simulink model "Quaternions_Method_merge_gio"  (R2021b)
settings: Solver=FixedStepAuto  StartTime=0.0  StopTime=Time  FixedStep=1e-3  RelTol=1e-13  AbsTol=1e-8
values from neighbouring files (symbols this model uses):
  a = 8.6251e+06    (= 8625100)    [Main.m]
  A_BN_0 = [1/3, 2/3, 2/3;             2/3, 1/3, -2/3;            -2/3, 2/3,-1/3]    [Main.m]
  A_rw = [1 0 0 1/sqrt(3);         0 1 0 1/sqrt(3) ... (first row only)    [Main.m]
  A_rw_star = [5/6 -1/6 -1/6;              -1/6  5/6 -1/6 ... (first row only)    [Main.m]
  c = 299792*10^3    (= 299792000)    [Main.m]
  e = 0.1195    [Main.m]
  f_mag = 5    [Main.m]
  G = [gn, gm, gvali, gsvi]    [Main.m]
  H = [hn, hm, hvali, hsvi]    [Main.m]
  H_0 = sqrt((g_1_0)^2 + (g_1_1)^2 + (h_1_1)^2)    [Main.m]
  i = 0.3815    [Main.m]
  MB = [2000; 0.3; 1; 0.12].*1e-2    [Main.m]
  mr = 1.2*1e-4    (= 0.00012)    [Main.m]
  muP = G*Mt    (= 398527110340000)    [Main.m]
  omega_0 = [om_x, om_y, om_z]    [Main.m]
  p_acc = deg2rad(5)    [Main.m]
  RD = 0.1*ones(1,10)    [Main.m]
  rho_d_MB = 0.1    [Main.m]
  rho_s_MB = 0.5    [Main.m]
  RS_MB = 0.5    [Main.m]
  RS_SP = 0.1    [Main.m]
  sig_b = sig_b^2    [Main.m]
  sig_n = 0.15*pi/180/3600/sqrt(t_sample)    [Main.m]
  SP = [2000; 0.3; 1; 0.12].*1e-2    [Main.m]
  T = 2*pi/n    [Main.m]
  t_sample = 1/5    (= 0.2)    [Main.m]
  theta0 = 0    [Main.m]
  w_E = (2*pi)/(24*3600)    (= 7.27220521664e-05)    [Main.m]
undefined symbols (not defined in the file or in its folder): magnitude
libraries: matrix_library x18, vrlib x8, simulink x2, simulink_extras x1
(part 5 of 6)

== system Quaternions_Method_merge_gio/Enviroment/Solar Radiation Perturbation/Torque_arm/creazione raggi vettore tra CM MB e centro facce illuminate della faccia che ha come normale l'asse j/If Action Subsystem1 ==
  Areas_vect : Inport
  MB : Inport  Port=2
  Action Port : ActionPort  ActionPortLabel=if(u1<0 & u2>0)
  Add : Sum  Inputs=+|-
  Add1 : Sum  Inputs=+|-
  Add2 : Sum
  Demux : Demux  Outputs=3
  Demux2 : Demux
  Divide : Product  Inputs=*/
  Divide1 : Product  Inputs=*/
  Gain{,1..3} (4 alike) : Gain  Gain=1/2
  Gain4 : Gain  Gain=-1
  Ground : Ground
  Ground1 : Ground
  Mux : Mux  Inputs=3
  Mux1 : Mux  Inputs=3
  Reshape : Reshape  OutputDimensionality=Column vector (2-D)
  Reshape2 : Reshape  OutputDimensionality=Column vector (2-D)
  Reshape3 : Reshape  OutputDimensionality=Column vector (2-D)
  Terminator{1..2,8..9} (4 alike) : Terminator
  r_cface_cluce_x_pos_z_neg : Outport
  wires:
  Demux/3 -> Terminator8/1
  Demux/1 -> Terminator9/1
  Add2/1 -> r_cface_cluce_x_pos_z_neg/1
  Reshape3/1 -> Add2/2
  Reshape2/1 -> Add2/1
  [a_MB] -> Gain2/1
  Divide1/1 -> Gain3/1
  Gain2/1 -> Add1/1
  Gain3/1 -> Add1/2
  Ground/1 -> Mux1/3, Mux1/2
  Mux1/1 -> Reshape3/1  "raggio vettore che collega il centro geom della faccia con il centro geom della faccia illuminata dal sole lungo i"
  [h_MB] -> Divide1/2
  Add1/1 -> Mux1/1
  Reshape/1 -> Demux/1
  Ground1/1 -> Mux/1, Mux/2
  Areas_vect/1 -> Reshape/1
  [a_MB] -> Divide/2
  Gain/1 -> Add/1
  [h_MB] -> Gain/1
  Demux/2 -> Divide/1, Divide1/1
  Gain1/1 -> Add/2
  Mux/1 -> Reshape2/1  "raggio vettore che collega il centro geom della faccia con il centro geom della faccia illuminata dal sole lungo -k"
  Divide/1 -> Gain1/1
  Add/1 -> Gain4/1
  Gain4/1 -> Mux/3
  Demux2/1 -> Terminator2/1
  Demux2/2 -> [a_MB]
  MB/1 -> Demux2/1
  Demux2/3 -> Terminator1/1
  Demux2/4 -> [h_MB]

== system Quaternions_Method_merge_gio/Enviroment/Solar Radiation Perturbation/Torque_arm/creazione raggi vettore tra CM MB e centro facce illuminate della faccia che ha come normale l'asse j/If Action Subsystem2 ==
  Areas_vect : Inport
  MB : Inport  Port=2
  Action Port : ActionPort  ActionPortLabel=if(u1>0 & u2<0)
  Add : Sum  Inputs=+|-
  Add1 : Sum  Inputs=+|-
  Add2 : Sum
  Demux : Demux  Outputs=3
  Demux2 : Demux
  Divide : Product  Inputs=*/
  Divide1 : Product  Inputs=*/
  Gain{,1..3} (4 alike) : Gain  Gain=1/2
  Gain4 : Gain  Gain=-1
  Ground : Ground
  Ground1 : Ground
  Mux : Mux  Inputs=3
  Mux1 : Mux  Inputs=3
  Reshape : Reshape  OutputDimensionality=Column vector (2-D)
  Reshape2 : Reshape  OutputDimensionality=Column vector (2-D)
  Reshape3 : Reshape  OutputDimensionality=Column vector (2-D)
  Terminator{1..2,8..9} (4 alike) : Terminator
  r_cface_cluce_x_neg_z_pos : Outport
  wires:
  Add/1 -> Mux/3
  Divide/1 -> Gain1/1
  Mux/1 -> Reshape2/1  "raggio vettore che collega il centro geom della faccia con il centro geom della faccia illuminata dal sole lungo k"
  Gain1/1 -> Add/2
  Demux/2 -> Divide1/1, Divide/1
  [h_MB] -> Gain/1
  Gain/1 -> Add/1
  [a_MB] -> Divide/2
  Areas_vect/1 -> Reshape/1
  Ground1/1 -> Mux/2, Mux/1
  Reshape/1 -> Demux/1
  [h_MB] -> Divide1/2
  Mux1/1 -> Reshape3/1  "raggio vettore che collega il centro geom della faccia con il centro geom della faccia illuminata dal sole lungo -i"
  Ground/1 -> Mux1/2, Mux1/3
  Gain3/1 -> Add1/2
  Gain2/1 -> Add1/1
  Divide1/1 -> Gain3/1
  [a_MB] -> Gain2/1
  Reshape2/1 -> Add2/1
  Reshape3/1 -> Add2/2
  Add2/1 -> r_cface_cluce_x_neg_z_pos/1
  Demux/1 -> Terminator9/1
  Demux/3 -> Terminator8/1
  Gain4/1 -> Mux1/1
  Add1/1 -> Gain4/1
  Demux2/1 -> Terminator2/1
  Demux2/2 -> [a_MB]
  MB/1 -> Demux2/1
  Demux2/3 -> Terminator1/1
  Demux2/4 -> [h_MB]

== system Quaternions_Method_merge_gio/Enviroment/Solar Radiation Perturbation/Torque_arm/creazione raggi vettore tra CM MB e centro facce illuminate della faccia che ha come normale l'asse j/If Action Subsystem3 ==
  Areas_vect : Inport
  MB : Inport  Port=2
  Action Port : ActionPort  ActionPortLabel=if(u1<0 & u2<0)
  Add : Sum  Inputs=+|-
  Add1 : Sum  Inputs=+|-
  Add2 : Sum
  Demux : Demux  Outputs=3
  Demux2 : Demux
  Divide : Product  Inputs=*/
  Divide1 : Product  Inputs=*/
  Gain{,1..3} (4 alike) : Gain  Gain=1/2
  Gain4 : Gain  Gain=-1
  Gain5 : Gain  Gain=-1
  Ground : Ground
  Ground1 : Ground
  Mux : Mux  Inputs=3
  Mux1 : Mux  Inputs=3
  Reshape : Reshape  OutputDimensionality=Column vector (2-D)
  Reshape2 : Reshape  OutputDimensionality=Column vector (2-D)
  Reshape3 : Reshape  OutputDimensionality=Column vector (2-D)
  Terminator{1..2,8..9} (4 alike) : Terminator
  r_cface_cluce_x_neg_z_neg : Outport
  wires:
  Add1/1 -> Gain4/1
  Gain4/1 -> Mux1/1
  Demux/3 -> Terminator8/1
  Demux/1 -> Terminator9/1
  Add2/1 -> r_cface_cluce_x_neg_z_neg/1
  Reshape3/1 -> Add2/2
  Reshape2/1 -> Add2/1
  [a_MB] -> Gain2/1
  Divide1/1 -> Gain3/1
  Gain2/1 -> Add1/1
  Gain3/1 -> Add1/2
  Ground/1 -> Mux1/3, Mux1/2
  Mux1/1 -> Reshape3/1  "raggio vettore che collega il centro geom della faccia con il centro geom della faccia illuminata dal sole lungo -i"
  [h_MB] -> Divide1/2
  Reshape/1 -> Demux/1
  Ground1/1 -> Mux/1, Mux/2
  Areas_vect/1 -> Reshape/1
  [a_MB] -> Divide/2
  Gain/1 -> Add/1
  [h_MB] -> Gain/1
  Demux/2 -> Divide/1, Divide1/1
  Gain1/1 -> Add/2
  Mux/1 -> Reshape2/1  "raggio vettore che collega il centro geom della faccia con il centro geom della faccia illuminata dal sole lungo -k"
  Divide/1 -> Gain1/1
  Add/1 -> Gain5/1
  Gain5/1 -> Mux/3
  Demux2/1 -> Terminator2/1
  Demux2/2 -> [a_MB]
  MB/1 -> Demux2/1
  Demux2/3 -> Terminator1/1
  Demux2/4 -> [h_MB]

== system Quaternions_Method_merge_gio/Enviroment/Solar Radiation Perturbation/Torque_arm/creazione raggi vettore tra CM MB e centro facce illuminate della faccia che ha come normale l'asse j/If Action Subsystem4 ==
  Action Port : ActionPort  ActionPortLabel=else
  Constant : Constant  Value=[0;0;0]
  Out1 : Outport
  wires:
  Constant/1 -> Out1/1

== system Quaternions_Method_merge_gio/Enviroment/Solar Radiation Perturbation/Torque_arm/creazione raggi vettore tra CM MB e centro facce illuminate della faccia che ha come normale l'asse j/If Action Subsystem5 ==
  Action Port : ActionPort  ActionPortLabel=else
  Constant : Constant  Value=[0;0;0]
  Out1 : Outport
  wires:
  Constant/1 -> Out1/1

== system Quaternions_Method_merge_gio/Enviroment/Solar Radiation Perturbation/Torque_arm/creazione raggi vettore tra CM MB e centro facce illuminate della faccia che ha come normale l'asse j/If Action Subsystem6 ==
  Action Port : ActionPort  ActionPortLabel=else
  Constant : Constant  Value=[0;0;0]
  Out1 : Outport
  wires:
  Constant/1 -> Out1/1

== system Quaternions_Method_merge_gio/Enviroment/Solar Radiation Perturbation/Torque_arm/creazione raggi vettore tra CM MB e centro facce illuminate della faccia che ha come normale l'asse j/If Action Subsystem7 ==
  Action Port : ActionPort  ActionPortLabel=else
  Constant : Constant  Value=[0;0;0]
  Out1 : Outport
  wires:
  Constant/1 -> Out1/1

== system Quaternions_Method_merge_gio/Enviroment/Solar Radiation Perturbation/Torque_arm/creazione raggi vettore tra CM MB e centro facce illuminate della faccia che ha come normale l'asse j/creating distance between cm MB and centro geom lato1 ==
  MB : Inport
  pointer : Inport  Port=2
  Demux : Demux
  Ground : Ground
  Mux : Mux  Inputs=3
  Product : Product
  Reshape : Reshape  OutputDimensionality=Column vector (2-D)
  Terminator : Terminator
  Terminator1 : Terminator
  Terminator2 : Terminator
  Out1 : Outport
  wires:
  Reshape/1 -> Out1/1
  Mux/1 -> Reshape/1
  MB/1 -> Demux/1
  Demux/1 -> Terminator/1
  Demux/2 -> Terminator1/1
  Demux/3 -> Terminator2/1
  Ground/1 -> Mux/2, Mux/1
  Demux/4 -> Product/1
  pointer/1 -> Product/2
  Product/1 -> Mux/3

== system Quaternions_Method_merge_gio/Enviroment/Solar Radiation Perturbation/Torque_arm/creazione raggi vettore tra CM MB e centro facce illuminate della faccia che ha come normale l'asse k/If Action Subsystem ==
  Areas_vect : Inport
  MB : Inport  Port=2
  Action Port : ActionPort  ActionPortLabel=if(u1>0 & u2>0)
  Add : Sum  Inputs=+|-
  Add1 : Sum  Inputs=+|-
  Add2 : Sum
  Demux : Demux  Outputs=3
  Demux1 : Demux  Outputs=3
  Demux2 : Demux
  Divide : Product  Inputs=*/
  Divide1 : Product  Inputs=*/
  Gain{,1..3} (4 alike) : Gain  Gain=1/2
  Ground : Ground
  Ground1 : Ground
  Mux : Mux  Inputs=3
  Mux1 : Mux  Inputs=3
  Reshape{,1..3} (4 alike) : Reshape  OutputDimensionality=Column vector (2-D)
  Terminator{,1..3,8..9} (6 alike) : Terminator
  r_cface_cluce_xy_pos : Outport
  wires:
  Add/1 -> Mux/2
  Divide/1 -> Gain1/1
  Mux/1 -> Reshape2/1  "raggio vettore che collega il centro geom della faccia con il centro geom della faccia illuminata dal sole lungo j"
  Gain1/1 -> Add/2
  Demux/3 -> Divide/1
  [b_MB] -> Gain/1
  Gain/1 -> Add/1
  [a_MB] -> Divide/2
  Areas_vect/1 -> Reshape/1, Reshape1/1
  Ground1/1 -> Mux/1, Mux/3
  Reshape/1 -> Demux/1
  Add1/1 -> Mux1/1
  [b_MB] -> Divide1/2
  Mux1/1 -> Reshape3/1  "raggio vettore che collega il centro geom della faccia con il centro geom della faccia illuminata dal sole lungo x"
  Ground/1 -> Mux1/2, Mux1/3
  Demux1/3 -> Divide1/1
  Gain3/1 -> Add1/2
  Gain2/1 -> Add1/1
  Reshape1/1 -> Demux1/1
  Divide1/1 -> Gain3/1
  [a_MB] -> Gain2/1
  Reshape2/1 -> Add2/1
  Reshape3/1 -> Add2/2
  Add2/1 -> r_cface_cluce_xy_pos/1
  Demux1/1 -> Terminator/1
  Demux1/2 -> Terminator1/1
  Demux/1 -> Terminator9/1
  Demux/2 -> Terminator8/1
  MB/1 -> Demux2/1
  Demux2/1 -> Terminator2/1
  Demux2/2 -> [a_MB]
  Demux2/3 -> [b_MB]
  Demux2/4 -> Terminator3/1

== system Quaternions_Method_merge_gio/Enviroment/Solar Radiation Perturbation/Torque_arm/creazione raggi vettore tra CM MB e centro facce illuminate della faccia che ha come normale l'asse k/If Action Subsystem1 ==
  Areas_vect : Inport
  MB : Inport  Port=2
  Action Port : ActionPort  ActionPortLabel=if(u1>0 & u2<0)
  Add : Sum  Inputs=+|-
  Add1 : Sum  Inputs=+|-
  Add2 : Sum
  Demux : Demux  Outputs=3
  Demux1 : Demux  Outputs=3
  Demux2 : Demux
  Divide : Product  Inputs=*/
  Divide1 : Product  Inputs=*/
  Gain{,1..3} (4 alike) : Gain  Gain=1/2
  Gain4 : Gain  Gain=-1
  Ground : Ground
  Ground1 : Ground
  Mux : Mux  Inputs=3
  Mux1 : Mux  Inputs=3
  Reshape{,1..3} (4 alike) : Reshape  OutputDimensionality=Column vector (2-D)
  Terminator{,1..3,8..9} (6 alike) : Terminator
  r_cface_cluce_xpos_y_neg : Outport
  wires:
  Add/1 -> Gain4/1
  Divide/1 -> Gain1/1
  Mux/1 -> Reshape2/1  "raggio vettore che collega il centro geom della faccia con il centro geom della faccia illuminata dal sole lungo -j"
  Gain1/1 -> Add/2
  Demux/3 -> Divide/1
  Gain/1 -> Add/1
  Areas_vect/1 -> Reshape/1, Reshape1/1
  Ground1/1 -> Mux/1, Mux/3
  Reshape/1 -> Demux/1
  Mux1/1 -> Reshape3/1  "raggio vettore che collega il centro geom della faccia con il centro geom della faccia illuminata dal sole lungo i"
  Ground/1 -> Mux1/2, Mux1/3
  Demux1/3 -> Divide1/1
  Gain3/1 -> Add1/2
  Gain2/1 -> Add1/1
  Reshape1/1 -> Demux1/1
  Divide1/1 -> Gain3/1
  Reshape2/1 -> Add2/1
  Reshape3/1 -> Add2/2
  Add2/1 -> r_cface_cluce_xpos_y_neg/1
  Demux1/1 -> Terminator/1
  Demux1/2 -> Terminator1/1
  Demux/1 -> Terminator9/1
  Demux/2 -> Terminator8/1
  Gain4/1 -> Mux/2
  [a_MB] -> Divide/2
  [b_MB] -> Gain/1
  Add1/1 -> Mux1/1
  [b_MB] -> Divide1/2
  [a_MB] -> Gain2/1
  Demux2/1 -> Terminator2/1
  Demux2/2 -> [a_MB]
  MB/1 -> Demux2/1
  Demux2/3 -> [b_MB]
  Demux2/4 -> Terminator3/1

== system Quaternions_Method_merge_gio/Enviroment/Solar Radiation Perturbation/Torque_arm/creazione raggi vettore tra CM MB e centro facce illuminate della faccia che ha come normale l'asse k/If Action Subsystem2 ==
  Areas_vect : Inport
  MB1 : Inport  Port=2
  Action Port : ActionPort  ActionPortLabel=if(u1<0 & u2<0)
  Add : Sum  Inputs=+|-
  Add1 : Sum  Inputs=+|-
  Add2 : Sum
  Demux : Demux  Outputs=3
  Demux1 : Demux  Outputs=3
  Demux2 : Demux
  Divide : Product  Inputs=*/
  Divide1 : Product  Inputs=*/
  Gain{,1..3} (4 alike) : Gain  Gain=1/2
  Gain4 : Gain  Gain=-1
  Gain5 : Gain  Gain=-1
  Ground : Ground
  Ground1 : Ground
  Mux : Mux  Inputs=3
  Mux1 : Mux  Inputs=3
  Reshape{,1..3} (4 alike) : Reshape  OutputDimensionality=Column vector (2-D)
  Terminator{,1..3,8..9} (6 alike) : Terminator
  r_cface_cluce_xneg_y_neg : Outport
  wires:
  [a_MB] -> Divide1/2
  [b_MB] -> Gain2/1
  Add1/1 -> Gain5/1
  Gain4/1 -> Mux/1
  Add/1 -> Gain4/1
  [a_MB] -> Gain/1
  [b_MB] -> Divide/2
  Divide/1 -> Gain1/1
  Mux/1 -> Reshape2/1  "raggio vettore che collega il centro geom della faccia con il centro geom della faccia illuminata dal sole lungo -i"
  Gain1/1 -> Add/2
  Demux/3 -> Divide/1
  Gain/1 -> Add/1
  Areas_vect/1 -> Reshape/1, Reshape1/1
  Ground1/1 -> Mux/3, Mux/2
  Reshape/1 -> Demux/1
  Mux1/1 -> Reshape3/1  "raggio vettore che collega il centro geom della faccia con il centro geom della faccia illuminata dal sole lungo -j"
  Ground/1 -> Mux1/3, Mux1/1
  Demux1/3 -> Divide1/1
  Gain3/1 -> Add1/2
  Gain2/1 -> Add1/1
  Reshape1/1 -> Demux1/1
  Divide1/1 -> Gain3/1
  Reshape2/1 -> Add2/1
  Reshape3/1 -> Add2/2
  Add2/1 -> r_cface_cluce_xneg_y_neg/1
  Demux1/1 -> Terminator/1
  Demux1/2 -> Terminator1/1
  Demux/1 -> Terminator9/1
  Demux/2 -> Terminator8/1
  Gain5/1 -> Mux1/2
  Demux2/1 -> Terminator2/1
  Demux2/2 -> [a_MB]
  MB1/1 -> Demux2/1
  Demux2/3 -> [b_MB]
  Demux2/4 -> Terminator3/1

== system Quaternions_Method_merge_gio/Enviroment/Solar Radiation Perturbation/Torque_arm/creazione raggi vettore tra CM MB e centro facce illuminate della faccia che ha come normale l'asse k/If Action Subsystem3 ==
  Action Port : ActionPort  ActionPortLabel=else
  Constant : Constant  Value=[0;0;0]
  Out1 : Outport
  wires:
  Constant/1 -> Out1/1

== system Quaternions_Method_merge_gio/Enviroment/Solar Radiation Perturbation/Torque_arm/creazione raggi vettore tra CM MB e centro facce illuminate della faccia che ha come normale l'asse k/If Action Subsystem4 ==
  Areas_vect : Inport
  MB1 : Inport  Port=2
  Action Port : ActionPort  ActionPortLabel=if(u1<0 & u2>0)
  Add : Sum  Inputs=+|-
  Add1 : Sum  Inputs=+|-
  Add2 : Sum
  Demux : Demux  Outputs=3
  Demux1 : Demux  Outputs=3
  Demux2 : Demux
  Divide : Product  Inputs=*/
  Divide1 : Product  Inputs=*/
  Gain{,1..3} (4 alike) : Gain  Gain=1/2
  Gain4 : Gain  Gain=-1
  Ground : Ground
  Ground1 : Ground
  Mux : Mux  Inputs=3
  Mux1 : Mux  Inputs=3
  Reshape{,1..3} (4 alike) : Reshape  OutputDimensionality=Column vector (2-D)
  Terminator{,1..3,8..9} (6 alike) : Terminator
  r_cface_cluce_xneg_y_pos : Outport
  wires:
  Demux/2 -> Terminator8/1
  Demux/1 -> Terminator9/1
  Demux1/2 -> Terminator1/1
  Demux1/1 -> Terminator/1
  Add2/1 -> r_cface_cluce_xneg_y_pos/1
  Reshape3/1 -> Add2/2
  Reshape2/1 -> Add2/1
  Divide1/1 -> Gain3/1
  Reshape1/1 -> Demux1/1
  Gain2/1 -> Add1/1
  Gain3/1 -> Add1/2
  Demux1/3 -> Divide1/1
  Ground/1 -> Mux1/1, Mux1/3
  Mux1/1 -> Reshape3/1  "raggio vettore che collega il centro geom della faccia con il centro geom della faccia illuminata dal sole lungo j"
  Reshape/1 -> Demux/1
  Ground1/1 -> Mux/2, Mux/3
  Areas_vect/1 -> Reshape1/1, Reshape/1
  Gain/1 -> Add/1
  Demux/3 -> Divide/1
  Gain1/1 -> Add/2
  Mux/1 -> Reshape2/1  "raggio vettore che collega il centro geom della faccia con il centro geom della faccia illuminata dal sole lungo -i"
  Divide/1 -> Gain1/1
  [b_MB] -> Divide/2
  [a_MB] -> Gain/1
  Add/1 -> Gain4/1
  Gain4/1 -> Mux/1
  Add1/1 -> Mux1/2
  [b_MB] -> Gain2/1
  [a_MB] -> Divide1/2
  Demux2/1 -> Terminator2/1
  Demux2/2 -> [a_MB]
  MB1/1 -> Demux2/1
  Demux2/3 -> [b_MB]
  Demux2/4 -> Terminator3/1

== system Quaternions_Method_merge_gio/Enviroment/Solar Radiation Perturbation/Torque_arm/creazione raggi vettore tra CM MB e centro facce illuminate della faccia che ha come normale l'asse k/If Action Subsystem5 ==
  Action Port : ActionPort  ActionPortLabel=else
  Constant : Constant  Value=[0;0;0]
  Out1 : Outport
  wires:
  Constant/1 -> Out1/1

== system Quaternions_Method_merge_gio/Enviroment/Solar Radiation Perturbation/Torque_arm/creazione raggi vettore tra CM MB e centro facce illuminate della faccia che ha come normale l'asse k/If Action Subsystem6 ==
  Action Port : ActionPort  ActionPortLabel=else
  Constant : Constant  Value=[0;0;0]
  Out1 : Outport
  wires:
  Constant/1 -> Out1/1

== system Quaternions_Method_merge_gio/Enviroment/Solar Radiation Perturbation/Torque_arm/creazione raggi vettore tra CM MB e centro facce illuminate della faccia che ha come normale l'asse k/If Action Subsystem7 ==
  Action Port : ActionPort  ActionPortLabel=else
  Constant : Constant  Value=[0;0;0]
  Out1 : Outport
  wires:
  Constant/1 -> Out1/1

== system Quaternions_Method_merge_gio/Enviroment/Solar Radiation Perturbation/Torque_arm/creazione raggi vettore tra CM MB e centro facce illuminate della faccia che ha come normale l'asse k/creating distance between cm MB and centro geom lato1 ==
  MB : Inport
  pointer : Inport  Port=2
  Demux : Demux
  Ground : Ground
  Mux : Mux  Inputs=3
  Product : Product
  Reshape : Reshape  OutputDimensionality=Column vector (2-D)
  Terminator : Terminator
  Terminator2 : Terminator
  Terminator3 : Terminator
  Out1 : Outport
  wires:
  Reshape/1 -> Out1/1
  Mux/1 -> Reshape/1
  MB/1 -> Demux/1
  Demux/1 -> Terminator/1
  Demux/3 -> Terminator2/1
  Ground/1 -> Mux/3, Mux/2
  Demux/4 -> Terminator3/1
  Product/1 -> Mux/1
  pointer/1 -> Product/2
  Demux/2 -> Product/1

== system Quaternions_Method_merge_gio/Sensors/Magnetometer1/Magnetometer /Error Matrices/A_NonOrtho ==
  Constant : Constant
  Constant1 : Constant  Value=0
  Constant2 : Constant  Value=0
  Constant3 : Constant  Value=-0.04
  Constant4 : Constant
  Constant5 : Constant  Value=0
  Constant6 : Constant  Value=0.02
  Constant7 : Constant  Value=0.01
  Constant8 : Constant
  Reshape : Reshape  OutputDimensionality=Customize  OutputDimensions=[3,3]
  Vector Concatenate : Concatenate  NumInputs=9
  A_no : Outport
  wires:
  [A31] -> Vector Concatenate/3
  [A12] -> Vector Concatenate/4
  [A21] -> Vector Concatenate/2
  [A33] -> Vector Concatenate/9
  [A32] -> Vector Concatenate/6
  [A22] -> Vector Concatenate/5
  [A13] -> Vector Concatenate/7
  [A23] -> Vector Concatenate/8
  [A11] -> Vector Concatenate/1
  Vector Concatenate/1 -> Reshape/1
  Reshape/1 -> A_no/1
  Constant/1 -> [A11]
  Constant1/1 -> [A21]
  Constant2/1 -> [A31]
  Constant3/1 -> [A12]
  Constant4/1 -> [A22]
  Constant5/1 -> [A32]
  Constant6/1 -> [A13]
  Constant7/1 -> [A23]
  Constant8/1 -> [A33]

== system Quaternions_Method_merge_gio/Sensors/Magnetometer1/Magnetometer /Error Matrices/A_ScaleFactor ==
  Constant : Constant  Value=1.08
  Constant{1..2,4..7} (6 alike) : Constant  Value=0
  Constant3 : Constant  Value=0.95
  Constant8 : Constant  Value=1.10
  Reshape : Reshape  OutputDimensionality=Customize  OutputDimensions=[3,3]
  Vector Concatenate : Concatenate  NumInputs=9
  A_sf : Outport
  wires:
  [A31] -> Vector Concatenate/3
  [A12] -> Vector Concatenate/4
  [A21] -> Vector Concatenate/2
  [A33] -> Vector Concatenate/9
  [A32] -> Vector Concatenate/6
  [A22] -> Vector Concatenate/5
  [A13] -> Vector Concatenate/7
  [A23] -> Vector Concatenate/8
  [A11] -> Vector Concatenate/1
  Vector Concatenate/1 -> Reshape/1
  Reshape/1 -> A_sf/1
  Constant/1 -> [A11]
  Constant1/1 -> [A21]
  Constant2/1 -> [A31]
  Constant4/1 -> [A12]
  Constant3/1 -> [A22]
  Constant5/1 -> [A32]
  Constant6/1 -> [A13]
  Constant7/1 -> [A23]
  Constant8/1 -> [A33]

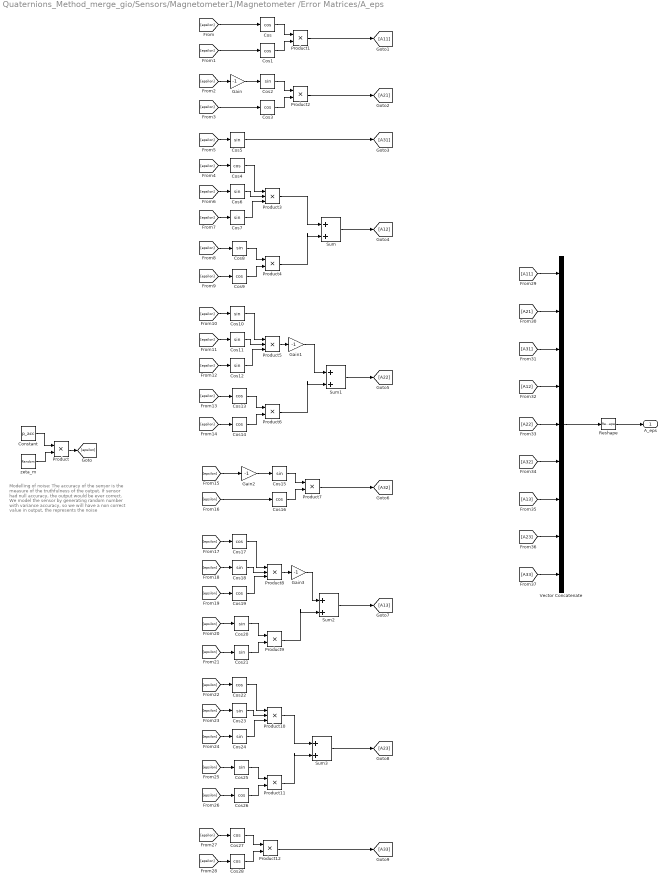
== system Quaternions_Method_merge_gio/Sensors/Magnetometer1/Magnetometer /Error Matrices/A_eps ==
  note: Modelling of noise: The accuracy of the sensor
      | is the measure of the truthfulness of the output.
      | If sensor had null accuracy, the output would be
      | ever correct. We model the  sensor by generating
      | random number with variance accuracy, so we
      | will have a non correct value in output, the
      | represents the noise
  Constant : Constant  Value=p_acc
  Cos{,1,3..4,9,13..14,16..17,19,22,26..28} (14 alike) : Trigonometry  Operator=cos
  Cos{2,5..8,10..12,15,18,20..21,23..25} (15 alike) : Trigonometry
  Gain{,1..3} (4 alike) : Gain  Gain=-1
  Product{,1..2,4,6..7,9,11..12} (9 alike) : Product
  Product{3,5,8,10} (4 alike) : Product  Inputs=3
  Reshape : Reshape  OutputDimensionality=Customize  OutputDimensions=[3,3]
  Sum{,1..3} (4 alike) : Sum  Inputs=|+|+|
  Vector Concatenate : Concatenate  NumInputs=9
  zeta_m : RandomNumber  Variance=p_acc  Seed=1  SampleTime=1/f_mag
  A_eps : Outport
  wires:
  Reshape/1 -> A_eps/1
  Vector Concatenate/1 -> Reshape/1
  Constant/1 -> Product/1
  zeta_m/1 -> Product/2
  Product/1 -> [epsilon]
  [epsilon] -> Cos/1
  [epsilon] -> Cos1/1
  Cos/1 -> Product1/1
  Cos1/1 -> Product1/2
  Product1/1 -> [A11]
  Cos2/1 -> Product2/1
  Cos3/1 -> Product2/2
  [epsilon] -> Cos3/1
  Product2/1 -> [A21]
  [epsilon] -> Gain/1
  Gain/1 -> Cos2/1
  [epsilon] -> Cos5/1
  Cos5/1 -> [A31]
  Cos4/1 -> Product3/1
  Cos6/1 -> Product3/2
  [epsilon] -> Cos4/1
  [epsilon] -> Cos6/1
  Product3/1 -> Sum/1
  [epsilon] -> Cos7/1
  Cos7/1 -> Product3/3
  [epsilon] -> Cos8/1
  Product4/1 -> Sum/2
  [epsilon] -> Cos9/1
  Cos9/1 -> Product4/2
  Cos8/1 -> Product4/1
  Sum/1 -> [A12]
  [epsilon] -> Cos11/1
  [epsilon] -> Cos10/1
  Cos11/1 -> Product5/2
  Cos10/1 -> Product5/1
  [epsilon] -> Cos13/1
  Sum1/1 -> [A22]
  Cos13/1 -> Product6/1
  [epsilon] -> Cos14/1
  Cos12/1 -> Product5/3
  Cos14/1 -> Product6/2
  Product6/1 -> Sum1/2
  [epsilon] -> Cos12/1
  Product5/1 -> Gain1/1
  Gain1/1 -> Sum1/1
  Gain2/1 -> Cos15/1
  [epsilon] -> Gain2/1
  Product7/1 -> [A32]
  Cos16/1 -> Product7/2
  Cos15/1 -> Product7/1
  [epsilon] -> Cos16/1
  Gain3/1 -> Sum2/1
  Product8/1 -> Gain3/1
  Cos18/1 -> Product8/2
  [epsilon] -> Cos18/1
  Sum2/1 -> [A13]
  Cos20/1 -> Product9/1
  Cos17/1 -> Product8/1
  [epsilon] -> Cos19/1
  Cos19/1 -> Product8/3
  Product9/1 -> Sum2/2
  [epsilon] -> Cos17/1
  Cos21/1 -> Product9/2
  [epsilon] -> Cos20/1
  [epsilon] -> Cos21/1
  [epsilon] -> Cos23/1
  [epsilon] -> Cos22/1
  Cos23/1 -> Product10/2
  Cos22/1 -> Product10/1
  [epsilon] -> Cos25/1
  Sum3/1 -> [A23]
  Cos25/1 -> Product11/1
  [epsilon] -> Cos26/1
  Product10/1 -> Sum3/1
  Cos24/1 -> Product10/3
  Cos26/1 -> Product11/2
  Product11/1 -> Sum3/2
  [epsilon] -> Cos24/1
  Cos27/1 -> Product12/1
  Cos28/1 -> Product12/2
  [epsilon] -> Cos27/1
  [epsilon] -> Cos28/1
  Product12/1 -> [A33]
  [A11] -> Vector Concatenate/1
  [A21] -> Vector Concatenate/2
  [A31] -> Vector Concatenate/3
  [A12] -> Vector Concatenate/4
  [A22] -> Vector Concatenate/5
  [A32] -> Vector Concatenate/6
  [A13] -> Vector Concatenate/7
  [A23] -> Vector Concatenate/8
  [A33] -> Vector Concatenate/9

== system Quaternions_Method_merge_gio/Sensors/Magnetometer1/b_B computation/Saturation/If Action Subsystem ==
  b_B : Inport
  Action Port : ActionPort  ActionPortLabel=if(u1 < mr)
  b_B* : Outport
  wires:
  b_B/1 -> b_B*/1

== system Quaternions_Method_merge_gio/Sensors/Magnetometer1/b_B computation/Saturation/If Action Subsystem1 ==
  mr : Inport
  b_B : Inport  Port=2
  Action Port : ActionPort  ActionPortLabel=else
  Normalize Vector : vrlib/Utilities/Normalize Vector  maxzero=0
  Product : Product
  b_B_sat : Outport
  wires:
  b_B/1 -> Normalize Vector/1
  Product/1 -> b_B_sat/1
  mr/1 -> Product/1
  Normalize Vector/1 -> Product/2

== system Quaternions_Method_merge_gio/Enviroment/Solar Radiation Perturbation/Sum forces/determine highlighted area/creazione della matrice che ha per colonne i vettori distanza tra il CM del MB e i centri geom delle aree illuminate dal sole /creazione raggi vettore tra CM MB e centro facce illuminate della faccia che ha come normale l'asse i ==
  S_B : Inport
  MB : Inport  Port=2
  A_vect : Inport  Port=3
  Add2 : Sum  Inputs=+|+|+|+|+
  Demux1 : Demux  Outputs=3
  If Action Subsystem : Subsystem  TreatAsAtomicUnit=on
  If Action Subsystem1 : Subsystem  TreatAsAtomicUnit=on
  If Action Subsystem2 : Subsystem  TreatAsAtomicUnit=on
  If Action Subsystem3 : Subsystem  TreatAsAtomicUnit=on
  If Action Subsystem4 : Subsystem  TreatAsAtomicUnit=on
  If Action Subsystem5 : Subsystem  TreatAsAtomicUnit=on
  If Action Subsystem6 : Subsystem  TreatAsAtomicUnit=on
  If Action Subsystem8 : Subsystem  TreatAsAtomicUnit=on
  If1 : If  NumInputs=2  IfExpression=u1>0 & u2>0
  If2 : If  NumInputs=2  IfExpression=u1<0 & u2>0
  If3 : If  NumInputs=2  IfExpression=u1>0 & u2<0
  If4 : If  NumInputs=2  IfExpression=u1<0 & u2<0
  Merge{,1..3} (4 alike) : Merge
  Reshape1 : Reshape  OutputDimensionality=Column vector (2-D)
  Terminator1 : Terminator
  creating distance between cm MB and centro geom lato : Subsystem
  Out1 : Outport
  wires:
  [A_vect] -> If Action Subsystem2/1(Areas_vect)
  [A_vect] -> If Action Subsystem1/1(Areas_vect)
  [A_vect] -> If Action Subsystem4/1(Areas_vect)
  Add2/1 -> Out1/1
  Merge3/1 -> Add2/5  "raggio vettore centro geom lato- centro geom lato illuminato"
  If4/1 -> If Action Subsystem2/Action
  If Action Subsystem2/1(r_cface_cluce_yneg_z_neg) -> Merge3/1
  If3/1 -> If Action Subsystem1/Action
  [A_vect] -> If Action Subsystem/1(Areas_vect)
  Merge1/1 -> Add2/3  "raggio vettore centro geom lato- centro geom lato illuminato"
  If Action Subsystem4/1(r_cface_cluce_zneg_y_pos) -> Merge1/1
  Merge/1 -> Add2/2  "raggio vettore centro geom lato- centro geom lato illuminato"
  If Action Subsystem/1(r_cface_cluce_yz_pos) -> Merge/1
  If1/2 -> If Action Subsystem8/Action
  S_B/1 -> Reshape1/1
  Reshape1/1 -> Demux1/1
  Demux1/2 -> If2/2, If3/2, If4/2, If1/2  "S_B_y"
  If2/1 -> If Action Subsystem4/Action
  If1/1 -> If Action Subsystem/Action
  Demux1/3 -> If4/1, If3/1, If2/1, If1/1  "S_B_z"
  creating distance between cm MB and centro geom lato/1(Out1) -> Add2/1
  Demux1/1 -> Terminator1/1  "S_B_x"
  MB/1 -> [MB]
  [MB] -> If Action Subsystem/2(MB)
  [MB] -> If Action Subsystem4/2(MB)
  [MB] -> If Action Subsystem1/2(MB)
  [MB] -> If Action Subsystem2/2(MB)
  If Action Subsystem8/1(Out1) -> Merge/2
  If2/2 -> If Action Subsystem3/Action
  If3/2 -> If Action Subsystem5/Action
  If4/2 -> If Action Subsystem6/Action
  If Action Subsystem3/1(Out1) -> Merge1/2
  If Action Subsystem1/1(r_cface_cluce_yneg_z_pos) -> Merge2/1
  If Action Subsystem5/1(Out1) -> Merge2/2
  Merge2/1 -> Add2/4  "raggio vettore centro geom lato- centro geom lato illuminato"
  If Action Subsystem6/1(Out1) -> Merge3/2
  [MB] -> creating distance between cm MB and centro geom lato/1(MB)
  A_vect/1 -> [A_vect]

== system Quaternions_Method_merge_gio/Enviroment/Solar Radiation Perturbation/Sum forces/determine highlighted area/creazione della matrice che ha per colonne i vettori distanza tra il CM del MB e i centri geom delle aree illuminate dal sole /creazione raggi vettore tra CM MB e centro facce illuminate della faccia che ha come normale l'asse j ==
  S_B : Inport
  MB : Inport  Port=2
  A_vect : Inport  Port=3
  Add2 : Sum  Inputs=+|+|+|+|+
  Demux1 : Demux  Outputs=3
  If Action Subsystem : Subsystem  TreatAsAtomicUnit=on
  If Action Subsystem1 : Subsystem  TreatAsAtomicUnit=on
  If Action Subsystem2 : Subsystem  TreatAsAtomicUnit=on
  If Action Subsystem3 : Subsystem  TreatAsAtomicUnit=on
  If Action Subsystem4 : Subsystem  TreatAsAtomicUnit=on
  If Action Subsystem5 : Subsystem  TreatAsAtomicUnit=on
  If Action Subsystem6 : Subsystem  TreatAsAtomicUnit=on
  If Action Subsystem7 : Subsystem  TreatAsAtomicUnit=on
  If1 : If  NumInputs=2  IfExpression=u1>0 & u2>0
  If2 : If  NumInputs=2  IfExpression=u1<0 & u2>0
  If3 : If  NumInputs=2  IfExpression=u1>0 & u2<0
  If4 : If  NumInputs=2  IfExpression=u1<0 & u2<0
  Merge{,1..3} (4 alike) : Merge
  Reshape1 : Reshape  OutputDimensionality=Column vector (2-D)
  Terminator1 : Terminator
  creating distance between cm MB and centro geom lato1 : Subsystem
  Out1 : Outport
  wires:
  Demux1/2 -> Terminator1/1
  creating distance between cm MB and centro geom lato1/1(Out1) -> Add2/1
  If1/1 -> If Action Subsystem/Action
  If2/1 -> If Action Subsystem1/Action
  Reshape1/1 -> Demux1/1
  S_B/1 -> Reshape1/1
  If Action Subsystem/1(r_cface_cluce_xz_pos) -> Merge/1
  Merge/1 -> Add2/2  "raggio vettore centro geom lato- centro geom lato illuminato"
  If Action Subsystem1/1(r_cface_cluce_x_pos_z_neg) -> Merge1/1
  Merge1/1 -> Add2/3  "raggio vettore centro geom lato- centro geom lato illuminato"
  [A_vect] -> If Action Subsystem/1(Areas_vect)
  Merge2/1 -> Add2/4  "raggio vettore centro geom lato- centro geom lato illuminato"
  If3/1 -> If Action Subsystem2/Action
  If Action Subsystem3/1(r_cface_cluce_x_neg_z_neg) -> Merge3/1
  If4/1 -> If Action Subsystem3/Action
  Merge3/1 -> Add2/5  "raggio vettore centro geom lato- centro geom lato illuminato"
  Add2/1 -> Out1/1
  [A_vect] -> If Action Subsystem1/1(Areas_vect)
  [A_vect] -> If Action Subsystem2/1(Areas_vect)
  [A_vect] -> If Action Subsystem3/1(Areas_vect)
  Demux1/3 -> If4/1, If3/1, If2/1, If1/1  "S_B_z"
  Demux1/1 -> If1/2, If4/2, If3/2, If2/2  "S_B_x"
  MB/1 -> [MB]
  [MB] -> If Action Subsystem/2(MB)
  [MB] -> If Action Subsystem1/2(MB)
  [MB] -> If Action Subsystem2/2(MB)
  [MB] -> If Action Subsystem3/2(MB)
  If1/2 -> If Action Subsystem5/Action
  If2/2 -> If Action Subsystem4/Action
  If3/2 -> If Action Subsystem6/Action
  If4/2 -> If Action Subsystem7/Action
  If Action Subsystem5/1(Out1) -> Merge/2
  If Action Subsystem4/1(Out1) -> Merge1/2
  If Action Subsystem2/1(r_cface_cluce_x_neg_z_pos) -> Merge2/1
  If Action Subsystem6/1(Out1) -> Merge2/2
  If Action Subsystem7/1(Out1) -> Merge3/2
  [MB] -> creating distance between cm MB and centro geom lato1/1(MB)
  A_vect/1 -> [A_vect]

== system Quaternions_Method_merge_gio/Enviroment/Solar Radiation Perturbation/Sum forces/determine highlighted area/creazione della matrice che ha per colonne i vettori distanza tra il CM del MB e i centri geom delle aree illuminate dal sole /creazione raggi vettore tra CM MB e centro facce illuminate della faccia che ha come normale l'asse k ==
  S_B : Inport
  MB : Inport  Port=2
  A_vect : Inport  Port=3
  Add2 : Sum  Inputs=+|+|+|+|+
  Demux1 : Demux  Outputs=3
  If Action Subsystem : Subsystem  TreatAsAtomicUnit=on
  If Action Subsystem1 : Subsystem  TreatAsAtomicUnit=on
  If Action Subsystem2 : Subsystem  TreatAsAtomicUnit=on
  If Action Subsystem3 : Subsystem  TreatAsAtomicUnit=on
  If Action Subsystem4 : Subsystem  TreatAsAtomicUnit=on
  If Action Subsystem5 : Subsystem  TreatAsAtomicUnit=on
  If Action Subsystem6 : Subsystem  TreatAsAtomicUnit=on
  If Action Subsystem7 : Subsystem  TreatAsAtomicUnit=on
  If1 : If  NumInputs=2  IfExpression=u1>0 & u2>0
  If2 : If  NumInputs=2  IfExpression=u1<0 & u2>0
  If3 : If  NumInputs=2  IfExpression=u1>0 & u2<0
  If4 : If  NumInputs=2  IfExpression=u1<0 & u2<0
  Merge{,1..3} (4 alike) : Merge
  Reshape1 : Reshape  OutputDimensionality=Column vector (2-D)
  Terminator1 : Terminator
  creating distance between cm MB and centro geom lato1 : Subsystem
  Out1 : Outport
  wires:
  Demux1/3 -> Terminator1/1
  Demux1/1 -> If1/1, If4/1, If3/1, If2/1  "S_B_x"
  If1/1 -> If Action Subsystem/Action
  If2/1 -> If Action Subsystem4/Action
  Demux1/2 -> If4/2, If3/2, If2/2, If1/2  "S_B_y"
  Reshape1/1 -> Demux1/1
  S_B/1 -> Reshape1/1
  If1/2 -> If Action Subsystem5/Action
  Merge/1 -> Add2/2  "raggio vettore centro geom lato- centro geom lato illuminato"
  Merge1/1 -> Add2/3  "raggio vettore centro geom lato- centro geom lato illuminato"
  [A_vect] -> If Action Subsystem/1(Areas_vect)
  Merge2/1 -> Add2/4  "raggio vettore centro geom lato- centro geom lato illuminato"
  If3/2 -> If Action Subsystem6/Action
  If Action Subsystem1/1(r_cface_cluce_xpos_y_neg) -> Merge2/1
  If3/1 -> If Action Subsystem1/Action
  If4/2 -> If Action Subsystem7/Action
  If4/1 -> If Action Subsystem2/Action
  Merge3/1 -> Add2/5  "raggio vettore centro geom lato- centro geom lato illuminato"
  Add2/1 -> Out1/1
  [A_vect] -> If Action Subsystem4/1(Areas_vect)
  [A_vect] -> If Action Subsystem1/1(Areas_vect)
  [A_vect] -> If Action Subsystem2/1(Areas_vect)
  MB/1 -> [MB]
  [MB] -> If Action Subsystem/2(MB)
  [MB] -> If Action Subsystem4/2(MB1)
  [MB] -> If Action Subsystem1/2(MB)
  [MB] -> If Action Subsystem2/2(MB1)
  If2/2 -> If Action Subsystem3/Action
  If Action Subsystem/1(r_cface_cluce_xy_pos) -> Merge/1
  If Action Subsystem5/1(Out1) -> Merge/2
  If Action Subsystem4/1(r_cface_cluce_xneg_y_pos) -> Merge1/1
  If Action Subsystem3/1(Out1) -> Merge1/2
  If Action Subsystem6/1(Out1) -> Merge2/2
  If Action Subsystem2/1(r_cface_cluce_xneg_y_neg) -> Merge3/1
  If Action Subsystem7/1(Out1) -> Merge3/2
  [MB] -> creating distance between cm MB and centro geom lato1/1(MB)
  creating distance between cm MB and centro geom lato1/1(Out1) -> Add2/1
  A_vect/1 -> [A_vect]

== system Quaternions_Method_merge_gio/Enviroment/Solar Radiation Perturbation/Sum forces/determine highlighted area/creazione della matrice che ha per colonne i vettori distanza tra il CM del MB e i centri geom delle aree illuminate dal sole /creazione raggi vettore tra CM MB e centro facce illuminate della faccia che ha come normale l'asse i/If Action Subsystem ==
  Areas_vect : Inport
  MB : Inport  Port=2
  Action Port : ActionPort  ActionPortLabel=if(u1>0 & u2>0)
  Add : Sum  Inputs=+|-
  Add1 : Sum  Inputs=+|-
  Add2 : Sum
  Demux : Demux  Outputs=3
  Demux2 : Demux
  Divide : Product  Inputs=*/
  Divide1 : Product  Inputs=*/
  Gain{,1..3} (4 alike) : Gain  Gain=1/2
  Ground : Ground
  Ground1 : Ground
  Mux : Mux  Inputs=3
  Mux1 : Mux  Inputs=3
  Reshape : Reshape  OutputDimensionality=Column vector (2-D)
  Reshape2 : Reshape  OutputDimensionality=Column vector (2-D)
  Reshape3 : Reshape  OutputDimensionality=Column vector (2-D)
  Terminator{1..2,8..9} (4 alike) : Terminator
  r_cface_cluce_yz_pos : Outport
  wires:
  Demux/2 -> Terminator8/1
  Demux/3 -> Terminator9/1
  Add2/1 -> r_cface_cluce_yz_pos/1
  Reshape3/1 -> Add2/2
  Reshape2/1 -> Add2/1
  [h_MB] -> Gain2/1
  Divide1/1 -> Gain3/1
  Gain2/1 -> Add1/1
  Gain3/1 -> Add1/2
  Ground/1 -> Mux1/2, Mux1/1
  Mux1/1 -> Reshape3/1  "raggio vettore che collega il centro geom della faccia con il centro geom della faccia illuminata dal sole lungo k"
  [b_MB] -> Divide1/2
  Reshape/1 -> Demux/1
  Ground1/1 -> Mux/3, Mux/1
  Areas_vect/1 -> Reshape/1
  [h_MB] -> Divide/2
  Gain/1 -> Add/1
  [b_MB] -> Gain/1
  Gain1/1 -> Add/2
  Mux/1 -> Reshape2/1  "raggio vettore che collega il centro geom della faccia con il centro geom della faccia illuminata dal sole lungo j"
  Divide/1 -> Gain1/1
  Demux/1 -> Divide1/1, Divide/1
  Add/1 -> Mux/2
  Add1/1 -> Mux1/3
  Demux2/1 -> Terminator2/1
  Demux2/2 -> Terminator1/1
  MB/1 -> Demux2/1
  Demux2/3 -> [b_MB]
  Demux2/4 -> [h_MB]

== system Quaternions_Method_merge_gio/Enviroment/Solar Radiation Perturbation/Sum forces/determine highlighted area/creazione della matrice che ha per colonne i vettori distanza tra il CM del MB e i centri geom delle aree illuminate dal sole /creazione raggi vettore tra CM MB e centro facce illuminate della faccia che ha come normale l'asse i/If Action Subsystem1 ==
  Areas_vect : Inport
  MB : Inport  Port=2
  Action Port : ActionPort  ActionPortLabel=if(u1>0 & u2<0)
  Add : Sum  Inputs=+|-
  Add1 : Sum  Inputs=+|-
  Add2 : Sum
  Demux : Demux  Outputs=3
  Demux2 : Demux
  Divide : Product  Inputs=*/
  Divide1 : Product  Inputs=*/
  Gain{,1..3} (4 alike) : Gain  Gain=1/2
  Gain4 : Gain  Gain=-1
  Ground : Ground
  Ground1 : Ground
  Mux : Mux  Inputs=3
  Mux1 : Mux  Inputs=3
  Reshape : Reshape  OutputDimensionality=Column vector (2-D)
  Reshape2 : Reshape  OutputDimensionality=Column vector (2-D)
  Reshape3 : Reshape  OutputDimensionality=Column vector (2-D)
  Terminator{1..2,8..9} (4 alike) : Terminator
  r_cface_cluce_yneg_z_pos : Outport
  wires:
  Add1/1 -> Mux1/3
  Demux/1 -> Divide/1, Divide1/1
  Divide/1 -> Gain1/1
  Mux/1 -> Reshape2/1  "raggio vettore che collega il centro geom della faccia con il centro geom della faccia illuminata dal sole lungo -j"
  Gain1/1 -> Add/2
  [b_MB] -> Gain/1
  Gain/1 -> Add/1
  [h_MB] -> Divide/2
  Areas_vect/1 -> Reshape/1
  Ground1/1 -> Mux/1, Mux/3
  Reshape/1 -> Demux/1
  [b_MB] -> Divide1/2
  Mux1/1 -> Reshape3/1  "raggio vettore che collega il centro geom della faccia con il centro geom della faccia illuminata dal sole lungo k"
  Ground/1 -> Mux1/1, Mux1/2
  Gain3/1 -> Add1/2
  Gain2/1 -> Add1/1
  Divide1/1 -> Gain3/1
  [h_MB] -> Gain2/1
  Reshape2/1 -> Add2/1
  Reshape3/1 -> Add2/2
  Add2/1 -> r_cface_cluce_yneg_z_pos/1
  Demux/3 -> Terminator9/1
  Demux/2 -> Terminator8/1
  Add/1 -> Gain4/1
  Gain4/1 -> Mux/2
  Demux2/1 -> Terminator2/1
  Demux2/2 -> Terminator1/1
  MB/1 -> Demux2/1
  Demux2/3 -> [b_MB]
  Demux2/4 -> [h_MB]

== system Quaternions_Method_merge_gio/Enviroment/Solar Radiation Perturbation/Sum forces/determine highlighted area/creazione della matrice che ha per colonne i vettori distanza tra il CM del MB e i centri geom delle aree illuminate dal sole /creazione raggi vettore tra CM MB e centro facce illuminate della faccia che ha come normale l'asse i/If Action Subsystem2 ==
  Areas_vect : Inport
  MB : Inport  Port=2
  Action Port : ActionPort  ActionPortLabel=if(u1<0 & u2<0)
  Add : Sum  Inputs=+|-
  Add1 : Sum  Inputs=+|-
  Add2 : Sum
  Demux : Demux  Outputs=3
  Demux2 : Demux
  Divide : Product  Inputs=*/
  Divide1 : Product  Inputs=*/
  Gain{,1..3} (4 alike) : Gain  Gain=1/2
  Gain4 : Gain  Gain=-1
  Gain5 : Gain  Gain=-1
  Ground : Ground
  Ground1 : Ground
  Mux : Mux  Inputs=3
  Mux1 : Mux  Inputs=3
  Reshape : Reshape  OutputDimensionality=Column vector (2-D)
  Reshape2 : Reshape  OutputDimensionality=Column vector (2-D)
  Reshape3 : Reshape  OutputDimensionality=Column vector (2-D)
  Terminator{1..2,8..9} (4 alike) : Terminator
  r_cface_cluce_yneg_z_neg : Outport
  wires:
  Gain4/1 -> Mux/2
  Add/1 -> Gain4/1
  Demux/2 -> Terminator8/1
  Demux/3 -> Terminator9/1
  Add2/1 -> r_cface_cluce_yneg_z_neg/1
  Reshape3/1 -> Add2/2
  Reshape2/1 -> Add2/1
  [h_MB] -> Gain2/1
  Divide1/1 -> Gain3/1
  Gain2/1 -> Add1/1
  Gain3/1 -> Add1/2
  Ground/1 -> Mux1/2, Mux1/1
  Mux1/1 -> Reshape3/1  "raggio vettore che collega il centro geom della faccia con il centro geom della faccia illuminata dal sole lungo -k"
  [b_MB] -> Divide1/2
  Reshape/1 -> Demux/1
  Ground1/1 -> Mux/3, Mux/1
  Areas_vect/1 -> Reshape/1
  [h_MB] -> Divide/2
  Gain/1 -> Add/1
  [b_MB] -> Gain/1
  Gain1/1 -> Add/2
  Mux/1 -> Reshape2/1  "raggio vettore che collega il centro geom della faccia con il centro geom della faccia illuminata dal sole lungo -j"
  Divide/1 -> Gain1/1
  Demux/1 -> Divide1/1, Divide/1
  Gain5/1 -> Mux1/3
  Add1/1 -> Gain5/1
  Demux2/1 -> Terminator2/1
  Demux2/2 -> Terminator1/1
  MB/1 -> Demux2/1
  Demux2/3 -> [b_MB]
  Demux2/4 -> [h_MB]

== system Quaternions_Method_merge_gio/Enviroment/Solar Radiation Perturbation/Sum forces/determine highlighted area/creazione della matrice che ha per colonne i vettori distanza tra il CM del MB e i centri geom delle aree illuminate dal sole /creazione raggi vettore tra CM MB e centro facce illuminate della faccia che ha come normale l'asse i/If Action Subsystem3 ==
  Action Port : ActionPort  ActionPortLabel=else
  Constant : Constant  Value=[0;0;0]
  Out1 : Outport
  wires:
  Constant/1 -> Out1/1

== system Quaternions_Method_merge_gio/Enviroment/Solar Radiation Perturbation/Sum forces/determine highlighted area/creazione della matrice che ha per colonne i vettori distanza tra il CM del MB e i centri geom delle aree illuminate dal sole /creazione raggi vettore tra CM MB e centro facce illuminate della faccia che ha come normale l'asse i/If Action Subsystem4 ==
  Areas_vect : Inport
  MB : Inport  Port=2
  Action Port : ActionPort  ActionPortLabel=if(u1<0 & u2>0)
  Add : Sum  Inputs=+|-
  Add1 : Sum  Inputs=+|-
  Add2 : Sum
  Demux : Demux  Outputs=3
  Demux2 : Demux
  Divide : Product  Inputs=*/
  Divide1 : Product  Inputs=*/
  Gain{,1..3} (4 alike) : Gain  Gain=1/2
  Gain4 : Gain  Gain=-1
  Ground : Ground
  Ground1 : Ground
  Mux : Mux  Inputs=3
  Mux1 : Mux  Inputs=3
  Reshape : Reshape  OutputDimensionality=Column vector (2-D)
  Reshape2 : Reshape  OutputDimensionality=Column vector (2-D)
  Reshape3 : Reshape  OutputDimensionality=Column vector (2-D)
  Terminator{1..2,8..9} (4 alike) : Terminator
  r_cface_cluce_zneg_y_pos : Outport
  wires:
  [h_MB] -> Divide1/2
  [b_MB] -> Gain2/1
  Add1/1 -> Mux1/2
  Gain4/1 -> Mux/3
  Add/1 -> Gain4/1
  [h_MB] -> Gain/1
  [b_MB] -> Divide/2
  Divide/1 -> Gain1/1
  Mux/1 -> Reshape2/1  "raggio vettore che collega il centro geom della faccia con il centro geom della faccia illuminata dal sole lungo -k"
  Gain1/1 -> Add/2
  Gain/1 -> Add/1
  Areas_vect/1 -> Reshape/1
  Ground1/1 -> Mux/1, Mux/2
  Reshape/1 -> Demux/1
  Mux1/1 -> Reshape3/1  "raggio vettore che collega il centro geom della faccia con il centro geom della faccia illuminata dal sole lungo j"
  Ground/1 -> Mux1/3, Mux1/1
  Gain3/1 -> Add1/2
  Gain2/1 -> Add1/1
  Divide1/1 -> Gain3/1
  Reshape2/1 -> Add2/1
  Reshape3/1 -> Add2/2
  Add2/1 -> r_cface_cluce_zneg_y_pos/1
  Demux/2 -> Terminator9/1
  Demux/3 -> Terminator8/1
  Demux/1 -> Divide1/1, Divide/1
  Demux2/1 -> Terminator2/1
  Demux2/2 -> Terminator1/1
  MB/1 -> Demux2/1
  Demux2/3 -> [b_MB]
  Demux2/4 -> [h_MB]

== system Quaternions_Method_merge_gio/Enviroment/Solar Radiation Perturbation/Sum forces/determine highlighted area/creazione della matrice che ha per colonne i vettori distanza tra il CM del MB e i centri geom delle aree illuminate dal sole /creazione raggi vettore tra CM MB e centro facce illuminate della faccia che ha come normale l'asse i/If Action Subsystem5 ==
  Action Port : ActionPort  ActionPortLabel=else
  Constant : Constant  Value=[0;0;0]
  Out1 : Outport
  wires:
  Constant/1 -> Out1/1

== system Quaternions_Method_merge_gio/Enviroment/Solar Radiation Perturbation/Sum forces/determine highlighted area/creazione della matrice che ha per colonne i vettori distanza tra il CM del MB e i centri geom delle aree illuminate dal sole /creazione raggi vettore tra CM MB e centro facce illuminate della faccia che ha come normale l'asse i/If Action Subsystem6 ==
  Action Port : ActionPort  ActionPortLabel=else
  Constant : Constant  Value=[0;0;0]
  Out1 : Outport
  wires:
  Constant/1 -> Out1/1

== system Quaternions_Method_merge_gio/Enviroment/Solar Radiation Perturbation/Sum forces/determine highlighted area/creazione della matrice che ha per colonne i vettori distanza tra il CM del MB e i centri geom delle aree illuminate dal sole /creazione raggi vettore tra CM MB e centro facce illuminate della faccia che ha come normale l'asse i/If Action Subsystem8 ==
  Action Port : ActionPort  ActionPortLabel=else
  Constant : Constant  Value=[0;0;0]
  Out1 : Outport
  wires:
  Constant/1 -> Out1/1

== system Quaternions_Method_merge_gio/Enviroment/Solar Radiation Perturbation/Sum forces/determine highlighted area/creazione della matrice che ha per colonne i vettori distanza tra il CM del MB e i centri geom delle aree illuminate dal sole /creazione raggi vettore tra CM MB e centro facce illuminate della faccia che ha come normale l'asse i/creating distance between cm MB and centro geom lato ==
  MB : Inport
  Demux : Demux
  Ground : Ground
  Mux : Mux  Inputs=3
  Reshape : Reshape  OutputDimensionality=Column vector (2-D)
  Terminator : Terminator
  Terminator1 : Terminator
  Terminator3 : Terminator
  Out1 : Outport
  wires:
  Reshape/1 -> Out1/1
  Mux/1 -> Reshape/1
  MB/1 -> Demux/1
  Demux/1 -> Terminator/1
  Demux/2 -> Terminator1/1
  Demux/3 -> Mux/2
  Ground/1 -> Mux/3, Mux/1
  Demux/4 -> Terminator3/1

== system Quaternions_Method_merge_gio/Enviroment/Solar Radiation Perturbation/Sum forces/determine highlighted area/creazione della matrice che ha per colonne i vettori distanza tra il CM del MB e i centri geom delle aree illuminate dal sole /creazione raggi vettore tra CM MB e centro facce illuminate della faccia che ha come normale l'asse j/If Action Subsystem ==
  Areas_vect : Inport
  MB : Inport  Port=2
  Action Port : ActionPort  ActionPortLabel=if(u1>0 & u2>0)
  Add : Sum  Inputs=+|-
  Add1 : Sum  Inputs=+|-
  Add2 : Sum
  Demux : Demux  Outputs=3
  Demux2 : Demux
  Divide : Product  Inputs=*/
  Divide1 : Product  Inputs=*/
  Gain{,1..3} (4 alike) : Gain  Gain=1/2
  Ground : Ground
  Ground1 : Ground
  Mux : Mux  Inputs=3
  Mux1 : Mux  Inputs=3
  Reshape : Reshape  OutputDimensionality=Column vector (2-D)
  Reshape2 : Reshape  OutputDimensionality=Column vector (2-D)
  Reshape3 : Reshape  OutputDimensionality=Column vector (2-D)
  Terminator{1..2,8..9} (4 alike) : Terminator
  r_cface_cluce_xz_pos : Outport
  wires:
  Add/1 -> Mux/3
  Divide/1 -> Gain1/1
  Mux/1 -> Reshape2/1  "raggio vettore che collega il centro geom della faccia con il centro geom della faccia illuminata dal sole lungo k"
  Gain1/1 -> Add/2
  Demux/2 -> Divide1/1, Divide/1
  [h_MB] -> Gain/1
  Gain/1 -> Add/1
  [a_MB] -> Divide/2
  Areas_vect/1 -> Reshape/1
  Ground1/1 -> Mux/2, Mux/1
  Reshape/1 -> Demux/1
  Add1/1 -> Mux1/1
  [h_MB] -> Divide1/2
  Mux1/1 -> Reshape3/1  "raggio vettore che collega il centro geom della faccia con il centro geom della faccia illuminata dal sole lungo i"
  Ground/1 -> Mux1/2, Mux1/3
  Gain3/1 -> Add1/2
  Gain2/1 -> Add1/1
  Divide1/1 -> Gain3/1
  [a_MB] -> Gain2/1
  Reshape2/1 -> Add2/1
  Reshape3/1 -> Add2/2
  Add2/1 -> r_cface_cluce_xz_pos/1
  Demux/1 -> Terminator9/1
  Demux/3 -> Terminator8/1
  Demux2/1 -> Terminator2/1
  Demux2/2 -> [a_MB]
  MB/1 -> Demux2/1
  Demux2/3 -> Terminator1/1
  Demux2/4 -> [h_MB]

== system Quaternions_Method_merge_gio/Enviroment/Solar Radiation Perturbation/Sum forces/determine highlighted area/creazione della matrice che ha per colonne i vettori distanza tra il CM del MB e i centri geom delle aree illuminate dal sole /creazione raggi vettore tra CM MB e centro facce illuminate della faccia che ha come normale l'asse j/If Action Subsystem1 ==
  Areas_vect : Inport
  MB : Inport  Port=2
  Action Port : ActionPort  ActionPortLabel=if(u1<0 & u2>0)
  Add : Sum  Inputs=+|-
  Add1 : Sum  Inputs=+|-
  Add2 : Sum
  Demux : Demux  Outputs=3
  Demux2 : Demux
  Divide : Product  Inputs=*/
  Divide1 : Product  Inputs=*/
  Gain{,1..3} (4 alike) : Gain  Gain=1/2
  Gain4 : Gain  Gain=-1
  Ground : Ground
  Ground1 : Ground
  Mux : Mux  Inputs=3
  Mux1 : Mux  Inputs=3
  Reshape : Reshape  OutputDimensionality=Column vector (2-D)
  Reshape2 : Reshape  OutputDimensionality=Column vector (2-D)
  Reshape3 : Reshape  OutputDimensionality=Column vector (2-D)
  Terminator{1..2,8..9} (4 alike) : Terminator
  r_cface_cluce_x_pos_z_neg : Outport
  wires:
  Demux/3 -> Terminator8/1
  Demux/1 -> Terminator9/1
  Add2/1 -> r_cface_cluce_x_pos_z_neg/1
  Reshape3/1 -> Add2/2
  Reshape2/1 -> Add2/1
  [a_MB] -> Gain2/1
  Divide1/1 -> Gain3/1
  Gain2/1 -> Add1/1
  Gain3/1 -> Add1/2
  Ground/1 -> Mux1/3, Mux1/2
  Mux1/1 -> Reshape3/1  "raggio vettore che collega il centro geom della faccia con il centro geom della faccia illuminata dal sole lungo i"
  [h_MB] -> Divide1/2
  Add1/1 -> Mux1/1
  Reshape/1 -> Demux/1
  Ground1/1 -> Mux/1, Mux/2
  Areas_vect/1 -> Reshape/1
  [a_MB] -> Divide/2
  Gain/1 -> Add/1
  [h_MB] -> Gain/1
  Demux/2 -> Divide/1, Divide1/1
  Gain1/1 -> Add/2
  Mux/1 -> Reshape2/1  "raggio vettore che collega il centro geom della faccia con il centro geom della faccia illuminata dal sole lungo -k"
  Divide/1 -> Gain1/1
  Add/1 -> Gain4/1
  Gain4/1 -> Mux/3
  Demux2/1 -> Terminator2/1
  Demux2/2 -> [a_MB]
  MB/1 -> Demux2/1
  Demux2/3 -> Terminator1/1
  Demux2/4 -> [h_MB]
